simulink model "PWM_Generator"  (R2014b)
settings: Solver=ode45  StartTime=0.0  StopTime=.3  MaxStep=.0001  RelTol=1e-3
values from neighbouring files (symbols this model uses):
  pwmResolution = 8    [motorParams.m]
libraries: simulink x1

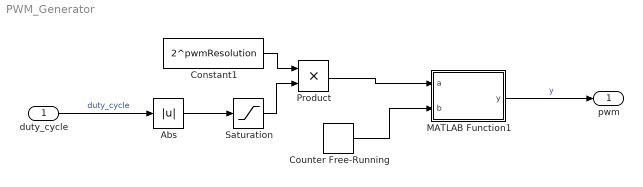
== system PWM_Generator ==
  duty_cycle : Inport  OutDataTypeStr=double  PortDimensions=1  SampleTime=0
  Abs : Abs
  Constant1 : Constant  Value=2^pwmResolution
  Counter Free-Running : simulink/Sources/Counter Free-Running  NumBits=pwmResolution  tsamp=pwmClockPeriod
  MATLAB Function1 : MATLAB Function  TreatAsAtomicUnit=on
      mask help: y = (a >= b) ? 1 : 0;
  Product : Product
  Saturation : Saturate  UpperLimit=1  LowerLimit=0
  pwm : Outport  OutDataTypeStr=double  PortDimensions=1  SampleTime=0
  wires:
  duty_cycle/1 -> Abs/1  "duty_cycle"
  Saturation/1 -> Product/2
  Counter Free-Running/1 -> MATLAB Function1/2(b)
  Constant1/1 -> Product/1
  Product/1 -> MATLAB Function1/1(a)
  MATLAB Function1/1(y) -> pwm/1  "y"
  Abs/1 -> Saturation/1

== matlab function PWM_Generator/MATLAB Function1 ==
function y = Comparator(a, b)
    if a>= b
        y = 1;
    else
        y = 0;
    end
